simulink model "inverted_pend_part1"  (R2019a)
settings: Solver=FixedStepAuto  StartTime=0.0  StopTime=5  FixedStep=0.01  RelTol=1e-3
values from neighbouring files (symbols this model uses):
  h = params.h    [prepare_sim.m]
  x0 = [0.2; 0]    [prepare_sim.m]
undefined symbols (not defined in the file or in its folder): stabilizing_mpc_controller
settings Model: Creator=Piku  LastModifiedBy=laperss

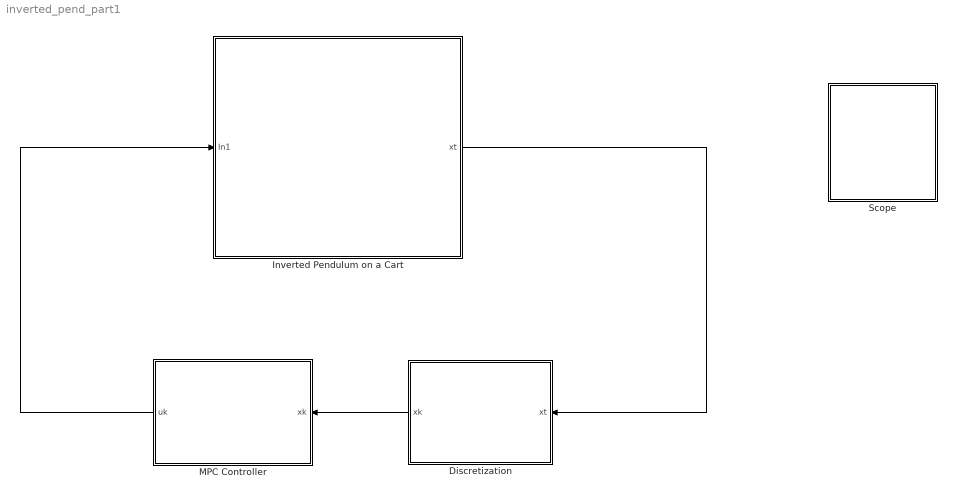
== system inverted_pend_part1 ==
  Discretization : Subsystem
  Inverted Pendulum on a Cart : Subsystem
      mask Display: image('cart_pendulum.png');
  MPC Controller : Subsystem
  Scope : Subsystem
  wires:
  Inverted Pendulum on a Cart/1("xt ") -> Discretization/1(xt)
  MPC Controller/1(uk) -> Inverted Pendulum on a Cart/1(In1)
  Discretization/1(xk) -> MPC Controller/1(" xk")

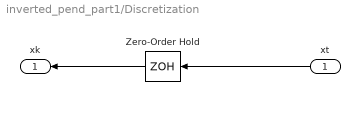
== system inverted_pend_part1/Discretization ==
  xt : Inport  PortDimensions=2
  Zero-Order Hold : ZeroOrderHold  SampleTime=h
  xk : Outport  PortDimensions=2
  wires:
  Zero-Order Hold/1 -> xk/1
  xt/1 -> Zero-Order Hold/1

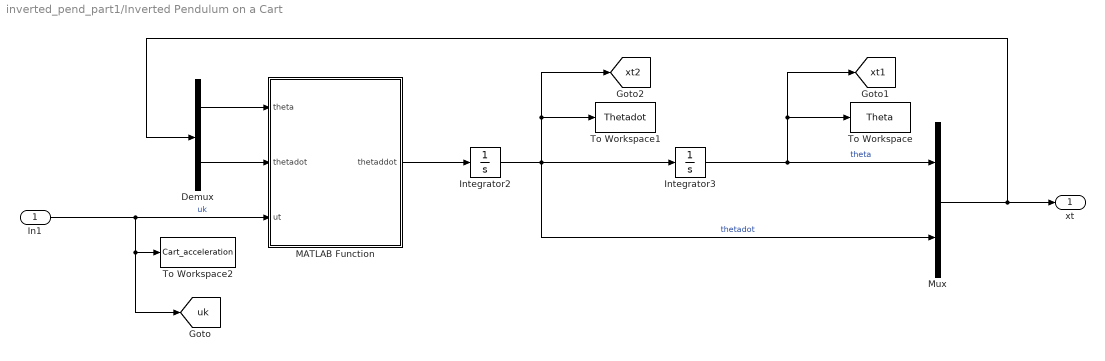
== system inverted_pend_part1/Inverted Pendulum on a Cart ==
  In1 : Inport  PortDimensions=1
  Demux : Demux  Outputs=2
  Integrator2 : Integrator  InitialCondition=x0(2)  UpperSaturationLimit=1e6  LowerSaturationLimit=-1e6
  Integrator3 : Integrator  InitialCondition=x0(1)  UpperSaturationLimit=pi  LowerSaturationLimit=-pi
  MATLAB Function : MATLAB Function  TreatAsAtomicUnit=on
  Mux : Mux  Inputs=2
  To Workspace : ToWorkspace  VariableName=Theta  SaveFormat=Timeseries  SampleTime=-1
  To Workspace1 : ToWorkspace  VariableName=Thetadot  SaveFormat=Timeseries  SampleTime=-1
  To Workspace2 : ToWorkspace  VariableName=Cart_acceleration  SaveFormat=Timeseries  SampleTime=-1
  "xt " : Outport  PortDimensions=2
  tag scope: uk=global, xt1=global, xt2=global
  wires:
  Integrator2/1 -> [xt2], To Workspace1/1, Mux/2, Integrator3/1  "thetadot"
  In1/1 -> MATLAB Function/3(ut), [uk], To Workspace2/1  "uk"
  Integrator3/1 -> Mux/1, To Workspace/1, [xt1]  "theta"
  Mux/1 -> Demux/1, "xt "/1
  MATLAB Function/1(thetaddot) -> Integrator2/1
  Demux/2 -> MATLAB Function/2(thetadot)
  Demux/1 -> MATLAB Function/1(theta)

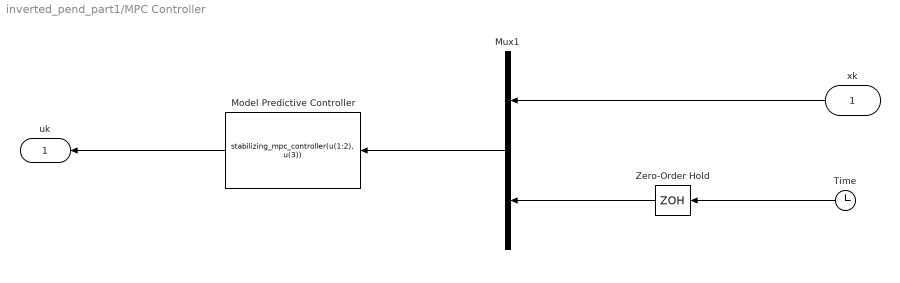
== system inverted_pend_part1/MPC Controller ==
  " xk" : Inport
  Model Predictive Controller : MATLABFcn  MATLABFcn=stabilizing_mpc_controller(u(1:2), u(3))  OutputDimensions=1
  Mux1 : Mux  Inputs=2
  Time : Clock
  Zero-Order Hold : ZeroOrderHold  SampleTime=-1
  uk : Outport
  wires:
  Mux1/1 -> Model Predictive Controller/1
  Model Predictive Controller/1 -> uk/1
  " xk"/1 -> Mux1/1
  Zero-Order Hold/1 -> Mux1/2
  Time/1 -> Zero-Order Hold/1

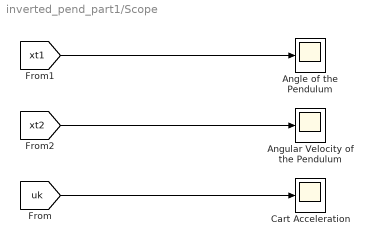
== system inverted_pend_part1/Scope ==
  Angle of the Pendulum : Scope
  Angular Velocity of the Pendulum : Scope
  Cart Acceleration : Scope
  wires:
  [xt1] -> Angle of the Pendulum/1
  [xt2] -> Angular Velocity of the Pendulum/1
  [uk] -> Cart Acceleration/1

== matlab function inverted_pend_part1/Inverted Pendulum on a Cart/MATLAB Function ==
  data: theta input; thetadot input; ut input; thetaddot output
function thetaddot = fcn(theta, thetadot, ut)
%% Parameters of the inverted pendulum
I   = 0.006;        % moment of inertia of the pendulum
m   = 0.2;          % Mass of the inverted pendulum
l   = 0.3;          % length to the pendulum center of mass
bp  = 0.012;        % coefficient of friction for pendulum
g   = 9.8;          % acceleration due to gravity

% Dynamics of the pendulum
a0 = -m*g*l/(I + m*l^2);
a1 = bp/(I + m*l^2);
b0 = m*l/(I + m*l^2);
thetaddot = -a0*sin(theta) -a1*thetadot + b0*cos(theta)*ut;
end
